simulink model "Horno_simulink"  (R2021a)
settings: Solver=VariableStepAuto  StartTime=0.0  StopTime=10.0  RelTol=1e-3
settings Model: Creator=Manu  LastModifiedBy=Manu

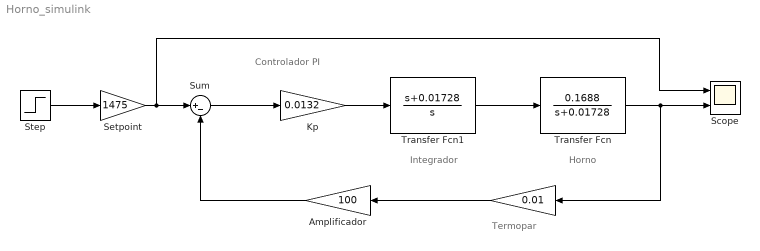
== system Horno_simulink ==
  note: Integrador
  note: Controlador PI
  note: Termopar
  note: Horno
  " " : Gain  Gain=0.01
  Amplificador : Gain  Gain=100
  Kp : Gain  Gain=0.0132
  Scope : Scope  NumInputPorts=2
  Setpoint : Gain  Gain=1475
  Step : Step  SampleTime=0
  Sum : Sum  Inputs=|+-
  Transfer Fcn : TransferFcn  Numerator=[0.1688]  Denominator=[1 0.01728]
  Transfer Fcn1 : TransferFcn  Numerator=[1 0.01728]  Denominator=[1 0]
  wires:
  Transfer Fcn1/1 -> Transfer Fcn/1
  Amplificador/1 -> Sum/2
  " "/1 -> Amplificador/1
  Transfer Fcn/1 -> " "/1, Scope/2
  Step/1 -> Setpoint/1
  Setpoint/1 -> Scope/1, Sum/1
  Kp/1 -> Transfer Fcn1/1
  Sum/1 -> Kp/1
